simulink model "Marine_LocoMotive_UAV_est_git"  (R2018a)
settings: Solver=ode4  StartTime=0.0  StopTime=40  FixedStep=T  MaxStep=2*T  MinStep=T  RelTol=1e-4
values from neighbouring files (symbols this model uses):
  a_11 = 0.05*m_b    (= 0.625)    [Marine_LocoMotive_UAV_est_git_parameters.m]    (also in Marine_LocoMotive_UAV_medium_est_git_parameters.m = 1.6875; heave_dynamics_chart.m)
  a_33 = m_b    (= 12.5)    [Marine_LocoMotive_UAV_est_git_parameters.m]    (also in Marine_LocoMotive_UAV_medium_est_git_parameters.m = 33.75; heave_dynamics_chart.m)
  A_w = 1*3.3/2    (= 1.65)    [Marine_LocoMotive_UAV_est_git_parameters.m]    (also in Marine_LocoMotive_UAV_medium_est_git_parameters.m = 0.6)
  A_w2 = 1*1.2/2    (= 0.6)    [Marine_LocoMotive_UAV_est_git_parameters.m]    (also in Marine_LocoMotive_UAV_medium_est_git_parameters.m = 0.305)
  Ac = 0.0331    [Marine_LocoMotive_UAV_est_git_parameters.m]    (also in Marine_LocoMotive_UAV_medium_est_git_parameters.m = 0.422)
  alpha_bar = pi/4    (= 0.785398163397)    [Marine_LocoMotive_UAV_est_git_parameters.m]    (also in Marine_LocoMotive_UAV_medium_est_git_parameters.m; heave_dynamics_chart.m = pi/4*sign(V_bar(j)))
  Am = sysd.denominator{1}    [Marine_LocoMotive_UAV_est_git_parameters.m]    (also in Marine_LocoMotive_UAV_medium_est_git_parameters.m)
  Am1_LPF = sysd.denominator{1}    [Marine_LocoMotive_UAV_est_git_parameters.m]    (also in Marine_LocoMotive_UAV_medium_est_git_parameters.m)
  Am2_LPF = sysd.denominator{1}    [Marine_LocoMotive_UAV_est_git_parameters.m]    (also in Marine_LocoMotive_UAV_medium_est_git_parameters.m)
  Am_asw_LPF = sysd.denominator{1}    [Marine_LocoMotive_UAV_est_git_parameters.m]    (also in Marine_LocoMotive_UAV_medium_est_git_parameters.m)
  Am_coup_LPF = sysd.denominator{1}    [Marine_LocoMotive_UAV_est_git_parameters.m]    (also in Marine_LocoMotive_UAV_medium_est_git_parameters.m)
  Am_fast_coup_LPF = sysd.denominator{1}    [Marine_LocoMotive_UAV_est_git_parameters.m]    (also in Marine_LocoMotive_UAV_medium_est_git_parameters.m)
  Am_rdeL_LPF = sysd.denominator{1}    [Marine_LocoMotive_UAV_est_git_parameters.m]    (also in Marine_LocoMotive_UAV_medium_est_git_parameters.m)
  Am_reL_LPF = sysd.denominator{1}    [Marine_LocoMotive_UAV_est_git_parameters.m]    (also in Marine_LocoMotive_UAV_medium_est_git_parameters.m)
  Am_rref20_LPF = sysd.denominator{1}    [Marine_LocoMotive_UAV_est_git_parameters.m]    (also in Marine_LocoMotive_UAV_medium_est_git_parameters.m)
  Am_rref_LPF = sysd.denominator{1}    [Marine_LocoMotive_UAV_est_git_parameters.m]    (also in Marine_LocoMotive_UAV_medium_est_git_parameters.m)
  AmAlpha_LPF = sysd.denominator{1}    [Marine_LocoMotive_UAV_est_git_parameters.m]    (also in Marine_LocoMotive_UAV_medium_est_git_parameters.m)
  Amp_sf = 3    [Marine_LocoMotive_UAV_est_git_parameters.m]    (also in Marine_LocoMotive_UAV_medium_est_git_parameters.m)
  Amp_sf_rp = 0.05*m_u*g    (= 0.8829)    [Marine_LocoMotive_UAV_est_git_parameters.m]    (also in Marine_LocoMotive_UAV_medium_est_git_parameters.m = 9.56475)
  AmV_LPF = sysd.denominator{1}    [Marine_LocoMotive_UAV_est_git_parameters.m]    (also in Marine_LocoMotive_UAV_medium_est_git_parameters.m)
  AmZ_LPF = sysd.denominator{1}    [Marine_LocoMotive_UAV_est_git_parameters.m]    (also in Marine_LocoMotive_UAV_medium_est_git_parameters.m)
  b_11 = 0    [Marine_LocoMotive_UAV_est_git_parameters.m]    (also in Marine_LocoMotive_UAV_medium_est_git_parameters.m; heave_dynamics_chart.m)
  b_33 = 2*m_b*omega_h    (= 19.6349540849)    [Marine_LocoMotive_UAV_est_git_parameters.m]    (also in Marine_LocoMotive_UAV_medium_est_git_parameters.m = 84.8230016469; buoyancy_calc.m = 4.18879020479; heave_dynamics_chart.m = 2*m_b*omega_h)
  Bm = sysd.numerator{1}    [Marine_LocoMotive_UAV_est_git_parameters.m]    (also in Marine_LocoMotive_UAV_medium_est_git_parameters.m)
  Bm1_LPF = sysd.numerator{1}    [Marine_LocoMotive_UAV_est_git_parameters.m]    (also in Marine_LocoMotive_UAV_medium_est_git_parameters.m)
  Bm2_LPF = sysd.numerator{1}    [Marine_LocoMotive_UAV_est_git_parameters.m]    (also in Marine_LocoMotive_UAV_medium_est_git_parameters.m)
  Bm_asw_LPF = sysd.numerator{1}    [Marine_LocoMotive_UAV_est_git_parameters.m]    (also in Marine_LocoMotive_UAV_medium_est_git_parameters.m)
  Bm_coup_LPF = sysd.numerator{1}    [Marine_LocoMotive_UAV_est_git_parameters.m]    (also in Marine_LocoMotive_UAV_medium_est_git_parameters.m)
  Bm_fast_coup_LPF = sysd.numerator{1}    [Marine_LocoMotive_UAV_est_git_parameters.m]    (also in Marine_LocoMotive_UAV_medium_est_git_parameters.m)
  Bm_rdeL_LPF = sysd.numerator{1}    [Marine_LocoMotive_UAV_est_git_parameters.m]    (also in Marine_LocoMotive_UAV_medium_est_git_parameters.m)
  Bm_reL_LPF = sysd.numerator{1}    [Marine_LocoMotive_UAV_est_git_parameters.m]    (also in Marine_LocoMotive_UAV_medium_est_git_parameters.m)
  Bm_rref20_LPF = sysd.numerator{1}    [Marine_LocoMotive_UAV_est_git_parameters.m]    (also in Marine_LocoMotive_UAV_medium_est_git_parameters.m)
  Bm_rref_LPF = sysd.numerator{1}    [Marine_LocoMotive_UAV_est_git_parameters.m]    (also in Marine_LocoMotive_UAV_medium_est_git_parameters.m)
  BmAlpha_LPF = sysd.numerator{1}    [Marine_LocoMotive_UAV_est_git_parameters.m]    (also in Marine_LocoMotive_UAV_medium_est_git_parameters.m)
  BmV_LPF = sysd.numerator{1}    [Marine_LocoMotive_UAV_est_git_parameters.m]    (also in Marine_LocoMotive_UAV_medium_est_git_parameters.m)
  BmZ_LPF = sysd.numerator{1}    [Marine_LocoMotive_UAV_est_git_parameters.m]    (also in Marine_LocoMotive_UAV_medium_est_git_parameters.m)
  C_S = [5;9]*10^-3    [Marine_LocoMotive_UAV_est_git_parameters.m]    (also in Marine_LocoMotive_UAV_medium_est_git_parameters.m; heave_dynamics_chart.m = 0.075/(log10(Re)-2)^2)
  Cd_u = 0.2    [Marine_LocoMotive_UAV_est_git_parameters.m]    (also in Marine_LocoMotive_UAV_medium_est_git_parameters.m)
  D_x = b_11 + D_s(1)    [Marine_LocoMotive_UAV_est_git_parameters.m]    (also in Marine_LocoMotive_UAV_medium_est_git_parameters.m; heave_dynamics_chart.m = b_11 + D_s(i,j))
  D_z = b_33 + D_s(2)    [Marine_LocoMotive_UAV_est_git_parameters.m]    (also in Marine_LocoMotive_UAV_medium_est_git_parameters.m; heave_dynamics_chart.m)
  dc_M_p = 6.7    [Marine_LocoMotive_UAV_est_git_parameters.m]    (also in Marine_LocoMotive_UAV_medium_est_git_parameters.m)
  Delta_h = (A_im/A_b-0.5)*h_b    (= -0.0625)    [Marine_LocoMotive_UAV_est_git_parameters.m]    (also in Marine_LocoMotive_UAV_medium_est_git_parameters.m = -0.075; heave_dynamics_chart.m)
  eps_V = 0.1    [Marine_LocoMotive_UAV_est_git_parameters.m]    (also in Marine_LocoMotive_UAV_medium_est_git_parameters.m)
  epsilon_1 = 5    [Marine_LocoMotive_UAV_est_git_parameters.m]    (also in Marine_LocoMotive_UAV_medium_est_git_parameters.m)
  epsilon_e_u1 = 0.05    [Marine_LocoMotive_UAV_est_git_parameters.m]    (also in Marine_LocoMotive_UAV_medium_est_git_parameters.m)
  epsilon_w = 0    [Marine_LocoMotive_UAV_est_git_parameters.m]    (also in Marine_LocoMotive_UAV_medium_est_git_parameters.m)
  epsilon_w2 = pi    (= 3.14159265359)    [Marine_LocoMotive_UAV_est_git_parameters.m]    (also in Marine_LocoMotive_UAV_medium_est_git_parameters.m)
  g = 9.81    [Marine_LocoMotive_UAV_est_git_parameters.m]    (also in Marine_LocoMotive_UAV_medium_est_git_parameters.m; heave_dynamics_chart.m)
  gamma_d_p = (2*0.3/0.03*2*0.2*12/4)/10    (= 2.4)    [Marine_LocoMotive_UAV_est_git_parameters.m]    (also in Marine_LocoMotive_UAV_medium_est_git_parameters.m)
  H = 10    [Marine_LocoMotive_UAV_est_git_parameters.m]    (also in Marine_LocoMotive_UAV_medium_est_git_parameters.m)
  h_b = 0.25    [Marine_LocoMotive_UAV_est_git_parameters.m]    (also in Marine_LocoMotive_UAV_medium_est_git_parameters.m = 0.3; buoyancy_calc.m = 0.15; heave_dynamics_chart.m)
  J_b = m_b*h_b*l_b/12    (= 0.208333333333)    [Marine_LocoMotive_UAV_est_git_parameters.m]    (also in Marine_LocoMotive_UAV_medium_est_git_parameters.m = 1.265625; heave_dynamics_chart.m)
  J_u = 0.03    [Marine_LocoMotive_UAV_est_git_parameters.m]    (also in Marine_LocoMotive_UAV_medium_est_git_parameters.m = 1.51708333333)
  K = 40    [Marine_LocoMotive_UAV_est_git_parameters.m]    (also in Marine_LocoMotive_UAV_medium_est_git_parameters.m = 83.3333333333)
  k3 = 24    [Marine_LocoMotive_UAV_est_git_parameters.m]    (also in Marine_LocoMotive_UAV_medium_est_git_parameters.m)
  k4 = 0.8    [Marine_LocoMotive_UAV_est_git_parameters.m]    (also in Marine_LocoMotive_UAV_medium_est_git_parameters.m)
  k_w = omega_w^2/g    (= 0.0628797426165)    [Marine_LocoMotive_UAV_est_git_parameters.m]    (also in Marine_LocoMotive_UAV_medium_est_git_parameters.m = 0.160972141098; heave_dynamics_chart.m = omega_w^2/g)
  k_w2 = omega_w2^2/g    (= 0.160972141098)    [Marine_LocoMotive_UAV_est_git_parameters.m]    (also in Marine_LocoMotive_UAV_medium_est_git_parameters.m = 0.251518970466)
  kd_a = 5.6    [Marine_LocoMotive_UAV_est_git_parameters.m]    (also in Marine_LocoMotive_UAV_medium_est_git_parameters.m)
  kd_r = 19.5    [Marine_LocoMotive_UAV_est_git_parameters.m]    (also in Marine_LocoMotive_UAV_medium_est_git_parameters.m)
  kd_t = 10    [Marine_LocoMotive_UAV_est_git_parameters.m]    (also in Marine_LocoMotive_UAV_medium_est_git_parameters.m = 25)
  kd_x = 5    [Marine_LocoMotive_UAV_est_git_parameters.m]    (also in Marine_LocoMotive_UAV_medium_est_git_parameters.m)
  kd_z = 2    [Marine_LocoMotive_UAV_est_git_parameters.m]    (also in Marine_LocoMotive_UAV_medium_est_git_parameters.m)
  ki_a = 1.6    [Marine_LocoMotive_UAV_est_git_parameters.m]    (also in Marine_LocoMotive_UAV_medium_est_git_parameters.m)
  ki_r = 9    [Marine_LocoMotive_UAV_est_git_parameters.m]    (also in Marine_LocoMotive_UAV_medium_est_git_parameters.m)
  ki_T = 12    [Marine_LocoMotive_UAV_est_git_parameters.m]    (also in Marine_LocoMotive_UAV_medium_est_git_parameters.m)
  ki_x = 1.2    [Marine_LocoMotive_UAV_est_git_parameters.m]    (also in Marine_LocoMotive_UAV_medium_est_git_parameters.m)
  ki_z = 1    [Marine_LocoMotive_UAV_est_git_parameters.m]    (also in Marine_LocoMotive_UAV_medium_est_git_parameters.m)
  kp_a = 9.6    [Marine_LocoMotive_UAV_est_git_parameters.m]    (also in Marine_LocoMotive_UAV_medium_est_git_parameters.m)
  kp_r = 45    [Marine_LocoMotive_UAV_est_git_parameters.m]    (also in Marine_LocoMotive_UAV_medium_est_git_parameters.m)
  kp_t = 20    [Marine_LocoMotive_UAV_est_git_parameters.m]    (also in Marine_LocoMotive_UAV_medium_est_git_parameters.m = 50)
  kp_T = 25    [Marine_LocoMotive_UAV_est_git_parameters.m]    (also in Marine_LocoMotive_UAV_medium_est_git_parameters.m)
  kp_x = 7    [Marine_LocoMotive_UAV_est_git_parameters.m]    (also in Marine_LocoMotive_UAV_medium_est_git_parameters.m)
  kp_z = 3    [Marine_LocoMotive_UAV_est_git_parameters.m]    (also in Marine_LocoMotive_UAV_medium_est_git_parameters.m)
  L = 0.2    [Marine_LocoMotive_UAV_est_git_parameters.m]    (also in Marine_LocoMotive_UAV_medium_est_git_parameters.m = 0.8)
  l_b = 0.8    [Marine_LocoMotive_UAV_est_git_parameters.m]    (also in Marine_LocoMotive_UAV_medium_est_git_parameters.m = 1.5; buoyancy_calc.m = 0.5; heave_dynamics_chart.m)
  Lc_0 = 7    [Marine_LocoMotive_UAV_est_git_parameters.m]    (also in Marine_LocoMotive_UAV_medium_est_git_parameters.m = 20)
  LIMIT_CMD_PITCH = 45*pi/180    (= 0.785398163397)    [Marine_LocoMotive_UAV_est_git_parameters.m]    (also in Marine_LocoMotive_UAV_medium_est_git_parameters.m)
  LIMIT_uCMD_HEIGHT = 0.9*n_motors*K    (= 144)    [Marine_LocoMotive_UAV_est_git_parameters.m]    (also in Marine_LocoMotive_UAV_medium_est_git_parameters.m = 450)
  m_b = rho_w*Vol_b/4    (= 12.5)    [Marine_LocoMotive_UAV_est_git_parameters.m]    (also in Marine_LocoMotive_UAV_medium_est_git_parameters.m = 33.75; buoyancy_calc.m = 5; heave_dynamics_chart.m)
  m_u = 1.8    [Marine_LocoMotive_UAV_est_git_parameters.m]    (also in Marine_LocoMotive_UAV_medium_est_git_parameters.m = 19.5)
  min_sf = 5    [Marine_LocoMotive_UAV_est_git_parameters.m]    (also in Marine_LocoMotive_UAV_medium_est_git_parameters.m)
  min_sf_rp = 0.35*m_u*g    (= 6.1803)    [Marine_LocoMotive_UAV_est_git_parameters.m]    (also in Marine_LocoMotive_UAV_medium_est_git_parameters.m = 66.95325)
  n_motors = 4    [Marine_LocoMotive_UAV_est_git_parameters.m]    (also in Marine_LocoMotive_UAV_medium_est_git_parameters.m = 6)
  nu_w = 1.787*10^-6    (= 1.787e-06)    [Marine_LocoMotive_UAV_est_git_parameters.m]    (also in Marine_LocoMotive_UAV_medium_est_git_parameters.m; buoyancy_calc.m; heave_dynamics_chart.m)
  omega_w = 2*pi/T_w    (= 0.785398163397)    [Marine_LocoMotive_UAV_est_git_parameters.m]    (also in Marine_LocoMotive_UAV_medium_est_git_parameters.m = 1.25663706144; heave_dynamics_chart.m = 2*pi/T_i)
  omega_w2 = 2*pi/T_w2    (= 1.25663706144)    [Marine_LocoMotive_UAV_est_git_parameters.m]    (also in Marine_LocoMotive_UAV_medium_est_git_parameters.m = 1.57079632679)
  r_0 = sqrt( (X0_b(1) - X0_u(1))^2 +(X0_b(2) - X0_u(2))^2 )    [Marine_LocoMotive_UAV_est_git_parameters.m]    (also in Marine_LocoMotive_UAV_medium_est_git_parameters.m)
  R_b = 0.1    [buoyancy_calc.m]
  r_bar = Lc_0-0.3    (= 6.7)    [Marine_LocoMotive_UAV_est_git_parameters.m]    (also in Marine_LocoMotive_UAV_medium_est_git_parameters.m = 19.7)
  r_min = (zu_bar-H)-0.2    [Marine_LocoMotive_UAV_est_git_parameters.m]    (also in Marine_LocoMotive_UAV_medium_est_git_parameters.m)
  rho_a = 1.225    [Marine_LocoMotive_UAV_est_git_parameters.m]    (also in Marine_LocoMotive_UAV_medium_est_git_parameters.m)
  rho_w = 1000    [Marine_LocoMotive_UAV_est_git_parameters.m]    (also in Marine_LocoMotive_UAV_medium_est_git_parameters.m; buoyancy_calc.m; heave_dynamics_chart.m)
  T = 1/500    (= 0.002)    [Marine_LocoMotive_UAV_est_git_parameters.m]    (also in Marine_LocoMotive_UAV_medium_est_git_parameters.m)
  T_init = 10    [Marine_LocoMotive_UAV_est_git_parameters.m]    (also in Marine_LocoMotive_UAV_medium_est_git_parameters.m)
  Theta0 = 0    [Marine_LocoMotive_UAV_est_git_parameters.m]    (also in Marine_LocoMotive_UAV_medium_est_git_parameters.m)
  torque_corr = 2*cosd(60)+1    [Marine_LocoMotive_UAV_est_git_parameters.m]    (also in Marine_LocoMotive_UAV_medium_est_git_parameters.m)
  u_s = w_dir*A_w^2*omega_w*k_w*exp(2*k_w*(-Delta_h/2))    [Marine_LocoMotive_UAV_est_git_parameters.m]    (also in Marine_LocoMotive_UAV_medium_est_git_parameters.m)
  u_s2 = w_dir2*A_w2^2*omega_w2*k_w2*exp(2*k_w2*(-Delta_h/2))    [Marine_LocoMotive_UAV_est_git_parameters.m]    (also in Marine_LocoMotive_UAV_medium_est_git_parameters.m)
  u_t = -1*0.5*1    (= -0.5)    [Marine_LocoMotive_UAV_est_git_parameters.m]    (also in Marine_LocoMotive_UAV_medium_est_git_parameters.m)
  u_w = 0*0.2    (= 0)    [Marine_LocoMotive_UAV_est_git_parameters.m]    (also in Marine_LocoMotive_UAV_medium_est_git_parameters.m)
  V0_b = [u_t+u_w+u_s+v_x_w, v_z_w].*[1 1]    [Marine_LocoMotive_UAV_est_git_parameters.m]    (also in Marine_LocoMotive_UAV_medium_est_git_parameters.m = [u_t+u_w+u_s+v_x_w, v_z_w])
  V0_u = V0_b    [Marine_LocoMotive_UAV_est_git_parameters.m]    (also in Marine_LocoMotive_UAV_medium_est_git_parameters.m = [0 0])
  V_bar = 4    [Marine_LocoMotive_UAV_est_git_parameters.m]    (also in Marine_LocoMotive_UAV_medium_est_git_parameters.m; heave_dynamics_chart.m = [-20:0.1:20]')
  Vol_b = A_b*l_b    (= 0.05)    [Marine_LocoMotive_UAV_est_git_parameters.m]    (also in Marine_LocoMotive_UAV_medium_est_git_parameters.m = 0.135; heave_dynamics_chart.m)
  w_dir = 1    [Marine_LocoMotive_UAV_est_git_parameters.m]    (also in Marine_LocoMotive_UAV_medium_est_git_parameters.m; heave_dynamics_chart.m)
  w_dir2 = 1    [Marine_LocoMotive_UAV_est_git_parameters.m]    (also in Marine_LocoMotive_UAV_medium_est_git_parameters.m)
  X0_b = [0,H-Delta_h]    [Marine_LocoMotive_UAV_est_git_parameters.m]    (also in Marine_LocoMotive_UAV_medium_est_git_parameters.m)
  X0_u = X0_b + [3/7 3/7]*Lc_0    [Marine_LocoMotive_UAV_est_git_parameters.m]    (also in Marine_LocoMotive_UAV_medium_est_git_parameters.m)
  zu_bar = X0_b(2) + Lc_0*sin(alpha_bar_0)    [Marine_LocoMotive_UAV_est_git_parameters.m]    (also in Marine_LocoMotive_UAV_medium_est_git_parameters.m)
undefined symbols (not defined in the file or in its folder): Am_HPF, Am_LPF, Am_LPF2, an1, an1_v, an2, an3, Bm_HPF, Bm_LPF, Bm_LPF2, bn1, bn1_v, bn2, bn3, DiscIntNeverNeededParam, F, Light, magnitude, MIL, OMEGA_FILTER_OUTER, Tc, Tg, Tn, Ts, Tsc, Tz, X_GPS_offset
libraries: simulink x55, simulink_extras x9, aerolibwind2 x2
(part 1 of 9)
settings Model: Creator=Ahmad  LastModifiedBy=Ahmad
settings SolverCC: InitialStep=T  AlgebraicLoopSolver=LineSearch

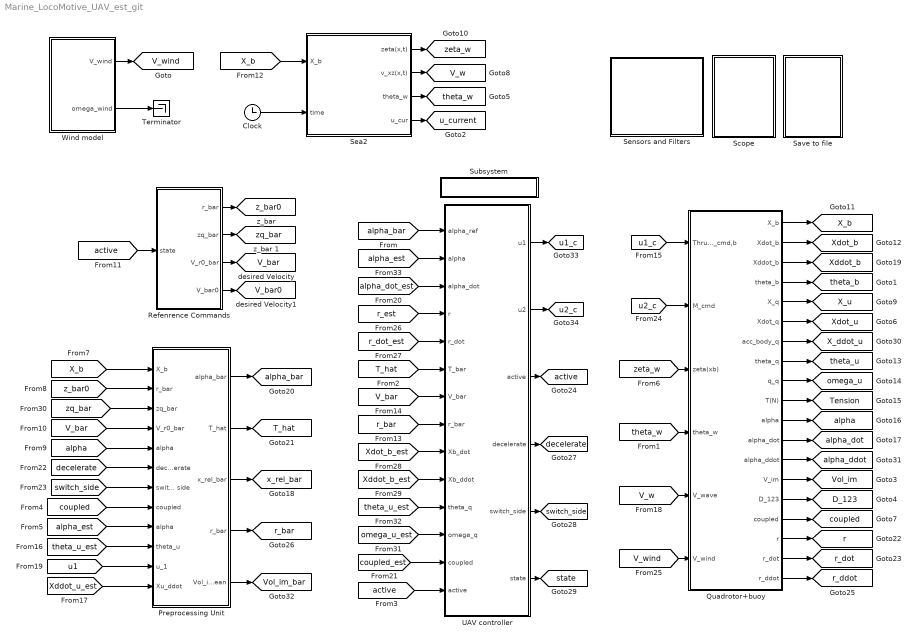
== system Marine_LocoMotive_UAV_est_git ==
  Clock : Clock
  Preprocessing Unit : Subsystem
  Quadrotor+buoy : Subsystem
  Refenrence Commands : Subsystem
  Save to file : Subsystem
  Scope : Subsystem
  Sea2 : Subsystem
  Sensors and Filters : Subsystem
  Subsystem : Subsystem
      settings: OpenFcn=Marine_LocoMotive_UAV_est_parameters
      mask Display:
      | text(.5,.5,'load parameters',...
      | 	'horizontalalignment','center');
  Terminator : Terminator
  UAV controller : Subsystem
  Wind model : Subsystem
  tag scope: D_123=global, T_hat=global, Tension=global, V_bar0=global, V_bar=global, V_w=global, V_wind=global, Vol_im=global, Vol_im_bar=global, X_b=global, X_ddot_u=global, X_u=global, Xddot_b=global, Xdot_b=global, Xdot_u=global, active=global, alpha=global, alpha_bar=global, alpha_ddot=global, alpha_dot=global, coupled=global, decelerate=global, omega_u=global, r=global, r_bar=global, r_ddot=global, r_dot=global, state=global, switch_side=global, theta_b=global, theta_u=global, theta_w=global, u1_c=global, u2_c=global, u_current=global, x_rel_bar=global, z_bar0=global, zeta_w=global, zq_bar=global
  wires:
  Clock/1 -> Sea2/2(time)
  [X_b] -> Sea2/1(X_b)
  Sea2/1(zeta(x,t)) -> [zeta_w]
  Sea2/2(v_xz(x,t)) -> [V_w]
  Sea2/3(theta_w) -> [theta_w]
  [theta_w] -> Quadrotor+buoy/4(theta_w)
  [V_w] -> Quadrotor+buoy/5(V_wave)
  [zeta_w] -> Quadrotor+buoy/3(zeta(xb))
  Quadrotor+buoy/5(X_q) -> [X_u]
  Quadrotor+buoy/1(X_b) -> [X_b]
  Quadrotor+buoy/2(Xdot_b) -> [Xdot_b]
  Quadrotor+buoy/8(theta_q) -> [theta_u]
  Quadrotor+buoy/9(q_q) -> [omega_u]
  Quadrotor+buoy/10(T(N)) -> [Tension]
  Quadrotor+buoy/11(alpha) -> [alpha]
  Quadrotor+buoy/12(alpha_dot) -> [alpha_dot]
  [X_b] -> Preprocessing Unit/1(X_b)
  Preprocessing Unit/1(alpha_bar) -> [alpha_bar]
  Preprocessing Unit/2(T_hat) -> [T_hat]
  Quadrotor+buoy/3(Xddot_b) -> [Xddot_b]
  Quadrotor+buoy/4(theta_b) -> [theta_b]
  Quadrotor+buoy/6(Xdot_q) -> [Xdot_u]
  Sea2/4(u_cur) -> [u_current]
  Quadrotor+buoy/14(V_im) -> [Vol_im]
  Quadrotor+buoy/15(D_123) -> [D_123]
  [alpha_bar] -> UAV controller/1(alpha_ref)
  [alpha_est] -> UAV controller/2(alpha)
  [alpha_dot_est] -> UAV controller/3(alpha_dot)
  [T_hat] -> UAV controller/6(T_bar)
  [V_bar] -> UAV controller/7(V_bar)
  [Xdot_b_est] -> UAV controller/9(Xb_dot)
  [Xddot_b_est] -> UAV controller/10(Xb_ddot)
  [theta_u_est] -> UAV controller/11(theta_q)
  [omega_u_est] -> UAV controller/12(omega_q)
  Quadrotor+buoy/16(coupled) -> [coupled]
  [active] -> Refenrence Commands/1(state)
  Preprocessing Unit/3(x_rel_bar) -> [x_rel_bar]
  [r_bar] -> UAV controller/8(r_bar)
  Quadrotor+buoy/17(r) -> [r]
  Quadrotor+buoy/18(r_dot) -> [r_dot]
  [r_est] -> UAV controller/4(r)
  UAV controller/3(" active") -> [active]
  [active] -> UAV controller/14(active)
  [coupled_est] -> UAV controller/13(coupled)
  Quadrotor+buoy/19(r_ddot) -> [r_ddot]
  [r_dot_est] -> UAV controller/5(r_dot)
  Preprocessing Unit/4(" r_bar") -> [r_bar]
  UAV controller/4(" decelerate") -> [decelerate]
  [decelerate] -> Preprocessing Unit/6(decelerate)
  UAV controller/5(" switch_side") -> [switch_side]
  UAV controller/6(state) -> [state]
  [switch_side] -> Preprocessing Unit/7(switch side)
  [alpha] -> Preprocessing Unit/5(alpha)
  [coupled] -> Preprocessing Unit/8(coupled)
  Quadrotor+buoy/7(acc_body_q) -> [X_ddot_u]
  Quadrotor+buoy/13(alpha_ddot) -> [alpha_ddot]
  [u1] -> Preprocessing Unit/11("u_1 ")
  [alpha_est] -> Preprocessing Unit/9("alpha ")
  [theta_u_est] -> Preprocessing Unit/10("theta_u ")
  [Xddot_u_est] -> Preprocessing Unit/12(Xu_ddot)
  Preprocessing Unit/5(Vol_im_mean) -> [Vol_im_bar]
  Wind model/1(V_wind) -> [V_wind]
  Wind model/2(omega_wind) -> Terminator/1
  [V_wind] -> Quadrotor+buoy/6(V_wind)
  Refenrence Commands/1(r_bar) -> [z_bar0]
  [z_bar0] -> Preprocessing Unit/2(r_bar)
  Refenrence Commands/4(V_bar0) -> [V_bar0]
  Refenrence Commands/3(V_r0_bar) -> [V_bar]
  [V_bar] -> Preprocessing Unit/4(V_r0_bar)
  UAV controller/1(u1) -> [u1_c]
  UAV controller/2(u2) -> [u2_c]
  [u1_c] -> Quadrotor+buoy/1(Thrust_cmd,b)
  [u2_c] -> Quadrotor+buoy/2(M_cmd)
  Refenrence Commands/2(zq_bar) -> [zq_bar]
  [zq_bar] -> Preprocessing Unit/3(zq_bar)

== system Marine_LocoMotive_UAV_est_git/Preprocessing Unit ==
  X_b : Inport
  r_bar : Inport  Port=2
  zq_bar : Inport  Port=3
  V_r0_bar : Inport  Port=4
  alpha : Inport  Port=5
  decelerate : Inport  Port=6
  switch side : Inport  Port=7
  coupled : Inport  Port=8
  "alpha " : Inport  Port=9
  "theta_u " : Inport  Port=10
  "u_1 " : Inport  Port=11
  Xu_ddot : Inport  Port=12
  Alpha_bar : Subsystem
  Buoy immersed volume estimation : Subsystem
  Discrete Transfer Fcn1 : DiscreteTransferFcn  Numerator=BmZ_LPF  Denominator=AmZ_LPF  InitialStates=[1 1]*(1-sum(AmZ_LPF))/(sum(BmZ_LPF))*X0_b(2)
  Mux : Mux  Inputs=3
  Sum : Sum  Inputs=|+-
  "T_bar " : Subsystem
  Terminator : Terminator
  "Theta_bar " : Subsystem
  V_r0_bar1 : InportShadow  Port=4
  buoy elvation : Scope
  r_bar1 : InportShadow  Port=2
  switch side1 : InportShadow  Port=7
  z_b : Selector  InputPortWidth=2  IndexOptions=Index vector (dialog)  Indices=2  OutputSizes=1
  alpha_bar : Outport
  T_hat : Outport  Port=2
  x_rel_bar : Outport  Port=3
  " r_bar" : Outport  Port=4
  Vol_im_mean : Outport  Port=5
  tag scope: T_bar=global, T_est=global, theta_bar=global, z_bar=global
  wires:
  X_b/1 -> z_b/1
  "Theta_bar "/1(theta_bar) -> "T_bar "/2(theta_bar), [theta_bar]
  V_r0_bar/1 -> "Theta_bar "/2(V_r0_bar)
  zq_bar/1 -> Alpha_bar/3(zq_bar)
  Mux/1 -> buoy elvation/1
  Sum/1 -> Mux/3
  z_b/1 -> Discrete Transfer Fcn1/1, Mux/1, Sum/1
  Discrete Transfer Fcn1/1 -> Mux/2, Sum/2, Alpha_bar/1(zb)  "better"
  [D11_bar] -> "Theta_bar "/3(D11_bar)
  Alpha_bar/1(alpha_bar) -> alpha_bar/1, "T_bar "/1("alpha_bar "), "Theta_bar "/1("alpha_bar ")
  "T_bar "/1(T_hat) -> T_hat/1
  "T_bar "/2(T_bar) -> [T_bar]
  r_bar/1 -> Alpha_bar/2(r_bar)
  Alpha_bar/2(x_rel_bar) -> x_rel_bar/1
  alpha/1 -> Alpha_bar/4(alpha)
  decelerate/1 -> Alpha_bar/5(decelerate)
  switch side/1 -> Alpha_bar/6(switch side)
  coupled/1 -> "T_bar "/4(coupled)
  switch side1/1 -> "Theta_bar "/4(switch side1)
  "theta_u "/1 -> "T_bar "/6(theta_u)
  "u_1 "/1 -> "T_bar "/7(u1)
  Xu_ddot/1 -> "T_bar "/8(Xu_ddot)
  "alpha "/1 -> "T_bar "/5(alpha)
  "T_bar "/3(T_est) -> [T_est]
  Alpha_bar/3(z_bar) -> [z_bar]
  Buoy immersed volume estimation/2(Vol_im_mean) -> Vol_im_mean/1
  V_r0_bar1/1 -> "T_bar "/3(V_r0_bar)
  r_bar1/1 -> " r_bar"/1
  Buoy immersed volume estimation/1(Vol_im_expected) -> Terminator/1
  "T_bar "/4(D_11_bar) -> [D11_bar]

== system Marine_LocoMotive_UAV_est_git/Quadrotor+buoy ==
  Thrust_cmd,b : Inport
  M_cmd : Inport  Port=2
  zeta(xb) : Inport  Port=3
  theta_w : Inport  Port=4
  V_wave : Inport  Port=5
  V_wind : Inport  Port=6
  3-DOF equations of motion Earth frame : Subsystem  mask(3DOF EoM, earth frame){pos_b_ini=X0_b, pos_u_ini=X0_u, theta_b_ini=0, alpha_0=alpha_bar, v_b_ini=V0_b, v_u_ini=V0_u, theta_q_ini=Theta0, q_b_ini=0, m_u=m_u, J_u=J_u, m_b=m_b, J_b=J_b, a_ii=[a_11 a_33], b_ii=[D_x,D_z], L=Lc_0, g=g, coupled_ini=off}
      mask prompts: pos_b_ini "Buoy initial position (x z):"; pos_u_ini "UAV initial position (x z):"; theta_b_ini "Buoy initial body attitude (quadrotor):"; alpha_0 "Cable initial angle:"; v_b_ini "Buoy initial velocity (x z):"; v_u_ini "UAV initial velocity (x z):"; theta_q_ini "Quadrotor initial body attitude (quadrotor):"; q_b_ini "Quadrotor initial body rotation rate:"; m_u "Quadrotor mass:"; J_u "Quadrotor moment of Inertia:"; m_b "Buoy mass:"; J_b "Buoy moment of Inertia:"; a_ii "Added mass (1x3):"; b_ii "Buoy damping coefficients (1x2):"; L "Cable length:"; g "gravity:"; coupled_ini "Initial coupling state (checked for coupled)"
      mask Display:
      | port_label('input',1,'u_1 (N)','texmode','on');
      | port_label('input',2,'u_2 (N.m)','texmode','on');
      | port_label('input',3,'\zeta (m)','texmode','on');
      | port_label('input',4,'\theta_w (rad)','texmode','on');
      | port_label('input',5,'V_{wave} (m/s)','texmode','on');
      | port_label('input',6,'V_{wind} (m/s)','texmode','on');
      | 
      | port_label('output',1,'X_b (m)','texmode','on');
      | port_label('output',2,'X_{b,dot} (m/s)','texmode','on');
      | port_label('output',3,'X_{b,ddot} (m/s)','texmode','on');
      | port_label('output',4,'\theta_b(rad)','texmode','on');
      | port_label('output',5,'X_q (m)','texmode','on');
      | port_label('output',6,'X_{q,dot} (m/s)','texmode','on');
      | port_label('output',7,'X_{q,ddot} (m/s^2)','texmode','on');
      | port_label('output',8,'\theta_q(rad)','texmode','on');
      | port_label('output',9,'\omega_q (rad/s)','texmode','on');
      | port_label('output',10,'\alpha (rad)','texmode','on');
      | port_label('output',11,'\alpha_{dot} (rad/s)','texmode','on');
      | port_label('output',12,'\alpha_{ddot} (rad/s)','texmode','on');
      | port_label('output',13,'r (m)','texmode','on');
      | port_label('output',14,'r_{dot} (m/s)','texmode','on');
      | port_label('output',15,'r_{ddot} (m/s)','texmode','on');
      | port_label('output',16,'T (N)','texmode','on');
      | port_label('output',17,'V_{im} (m^3)','texmode','on');
      | port_label('output',18,'D_{123}','texmode','on');
      | port_label('output',19,'coupled','texmode','on');
  Gain : Gain
  Gain1 : Gain
  Mux : Mux  Inputs=2
  Mux1 : Mux  Inputs=2
  Saturation - Limit Height Controller1 : Saturate  UpperLimit=K*L*torque_corr  LowerLimit=-K*L*torque_corr
  Saturation - Limit Height Controller3 : Saturate  UpperLimit=n_motors*K  LowerLimit=0
  Torque : Scope
  "Xb " : Scope
  "Xq " : Scope
  motor dynamics (thrust) : DiscreteTransferFcn  Numerator=Bm  Denominator=Am  InitialStates=-Am(2)/Bm(2)*m_u*g/cos(Theta0)
  motor dynamics (torque) : DiscreteTransferFcn  Numerator=Bm  Denominator=Am
  thrust : Scope
  X_b : Outport
  Xdot_b : Outport  Port=2
  Xddot_b : Outport  Port=3
  theta_b : Outport  Port=4
  X_q : Outport  Port=5
  Xdot_q : Outport  Port=6
  acc_body_q : Outport  Port=7
  theta_q : Outport  Port=8
  q_q : Outport  Port=9
  T(N) : Outport  Port=10
  alpha : Outport  Port=11
  alpha_dot : Outport  Port=12
  alpha_ddot : Outport  Port=13
  V_im : Outport  Port=14
  D_123 : Outport  Port=15
  coupled : Outport  Port=16
  r : Outport  Port=17
  r_dot : Outport  Port=18
  r_ddot : Outport  Port=19
  tag scope: u1=global, u2=global
  wires:
  Saturation - Limit Height Controller3/1 -> Gain/1, Mux/2
  motor dynamics (torque)/1 -> Saturation - Limit Height Controller1/1
  M_cmd/1 -> Mux1/1, motor dynamics (torque)/1
  Thrust_cmd,b/1 -> Mux/1, motor dynamics (thrust)/1
  Saturation - Limit Height Controller1/1 -> Mux1/2, Gain1/1
  zeta(xb)/1 -> 3-DOF equations of motion Earth frame/3(zeta)
  theta_w/1 -> 3-DOF equations of motion Earth frame/4(theta_w)
  V_wave/1 -> 3-DOF equations of motion Earth frame/5(V_w)
  3-DOF equations of motion Earth frame/5(Xu) -> "Xq "/1, X_q/1  "X_q"
  3-DOF equations of motion Earth frame/1(Xb) -> "Xb "/1, X_b/1  "X_b"
  3-DOF equations of motion Earth frame/2(Xb_dot) -> Xdot_b/1  "Xdot_b"
  3-DOF equations of motion Earth frame/6(Xu_dot) -> Xdot_q/1  "V_q"
  3-DOF equations of motion Earth frame/4(Attitude_buoy) -> theta_b/1  "theta_b"
  3-DOF equations of motion Earth frame/8(Attitude_quadrotor) -> theta_q/1  "theta_q"
  3-DOF equations of motion Earth frame/9(q_quadrotor) -> q_q/1  "omega_q"
  3-DOF equations of motion Earth frame/3(Xb_ddot) -> Xddot_b/1
  motor dynamics (thrust)/1 -> Saturation - Limit Height Controller3/1
  3-DOF equations of motion Earth frame/11(alpha_dot) -> alpha_dot/1  "alpha_dot"
  3-DOF equations of motion Earth frame/16(Cable Tension) -> T(N)/1  "tension"
  3-DOF equations of motion Earth frame/10(alpha) -> alpha/1  "alpha"
  Mux/1 -> thrust/1
  Mux1/1 -> Torque/1
  3-DOF equations of motion Earth frame/17(V_im) -> V_im/1
  Gain/1 -> 3-DOF equations of motion Earth frame/1(u1), [u1]
  Gain1/1 -> [u2], 3-DOF equations of motion Earth frame/2(u2)
  3-DOF equations of motion Earth frame/18("D_123 ") -> D_123/1
  3-DOF equations of motion Earth frame/19(coupled) -> coupled/1
  3-DOF equations of motion Earth frame/13("  r") -> r/1
  3-DOF equations of motion Earth frame/14("  rdot") -> r_dot/1
  3-DOF equations of motion Earth frame/15("  rddot") -> r_ddot/1
  3-DOF equations of motion Earth frame/7(Xu_ddot) -> acc_body_q/1
  3-DOF equations of motion Earth frame/12(alpha_ddot) -> alpha_ddot/1
  V_wind/1 -> 3-DOF equations of motion Earth frame/6(V_wind)

== system Marine_LocoMotive_UAV_est_git/Refenrence Commands ==
  note: Smooth reference signals
  note: Initialization phase, reference r and zu
  note: Saturation protection
  note: V_r0_bar is the velocity of the buoy relative
      | to the water current (wave velocity is not included)
  note: Refecence velocity
  state : Inport
  "  Vbar  " : Scope
  "  c" : Scope
  Bias : Bias  Bias=H+h_b/2
  Bias1 : Bias  Bias=-H-h_b/2
  Constant : Constant  Value=H
  Discrete Transfer Fcn (with initial outputs)1 : simulink_extras/Additional Discrete/Discrete Transfer Fcn (with initial outputs)  N=Bm_rref_LPF  D=Am_rref_LPF  U0=0  Y0=r_0  TS=-1
      settings: SourceProductName=Simulink  SourceProductBaseCode=SL
  Discrete Transfer Fcn (with initial outputs)3 : simulink_extras/Additional Discrete/Discrete Transfer Fcn (with initial outputs)  N=BmV_LPF  D=AmV_LPF  U0=0  Y0=0  TS=-1
      settings: SourceProductName=Simulink  SourceProductBaseCode=SL
  Discrete Transfer Fcn (with initial outputs)4 : simulink_extras/Additional Discrete/Discrete Transfer Fcn (with initial outputs)  N=Bm_rref20_LPF  D=Am_rref20_LPF  U0=0  Y0=r_0  TS=-1
      settings: SourceProductName=Simulink  SourceProductBaseCode=SL
  From File : FromFile  Commented=on  FileName=Export\with waves\SVC\V_bar.mat  SampleTime=0
  From File1 : FromFile  Commented=on  FileName=Export\no waves\SVC\V_bar.mat  SampleTime=0
  From File2 : FromFile  FileName=Export\Monte Carlo\CM_21\SVCS\V_bar.mat  SampleTime=0
  Gain : Gain  Gain=0
  Manual Switch1 : ManualSwitch  CurrentSetting=0
  Manual Switch2 : ManualSwitch  Commented=on
  Manual Switch3 : ManualSwitch
  Manual Switch4 : ManualSwitch
  Mux3 : Mux  Inputs=3
  "Rate Limiter for fly over test " : RateLimiter  RisingSlewLimit=2.5/10  FallingSlewLimit=-2.5/10  SampleTimeMode=inherited
  Saturation Dynamic : simulink/Discontinuities/Saturation Dynamic  OutMin=[]  OutMax=[]  OutDataTypeStr=Inherit: Same as second input  OutDataType=fixdt(1, 16)  OutScaling=2^-10  DoSatur=off
  Saturation Dynamic1 : simulink/Discontinuities/Saturation Dynamic  OutMin=[]  OutMax=[]  OutDataTypeStr=Inherit: Same as second input  OutDataType=fixdt(1, 16)  OutScaling=2^-10  DoSatur=off
  Selector1 : Selector  InputPortWidth=2  IndexOptions=Index vector (dialog)  Indices=1  OutputSizes=1
  Step : Step  Time=T_init  After=V_bar+1  SampleTime=0
  Step1 : Step  Time=T_init+25  After=V_bar+1  SampleTime=0
  Step3 : Step  Time=T_init+25+20  After=V_bar  SampleTime=0
  Step5 : Step  Commented=on  Time=T_init+20  After=-20  SampleTime=0
  Step6 : Step  Time=T_init  After=20  SampleTime=0
  Sum : Sum  Inputs=+--
  Sum2 : Sum  Inputs=|++
  Switch{,1..2,4} (4 alike) : Switch  Criteria=u2 > Threshold
  cable length : Constant  Value=Lc_0
  initialize : Step  SampleTime=0
  initialize r_bar : Step  Time=20  SampleTime=0
  minimum velocity error : Constant
  r error threshold [m] : Constant  Value=0.05
  r_bar_0 : Constant  Value=r_0
  "r_ref " : Constant  Value=r_bar
  r_ref for the coupled case (pulling) : Constant  Value=Lc_0
  setpoint velocity controller : MATLAB Function  TreatAsAtomicUnit=on
  smooth z_bar : simulink_extras/Additional Discrete/Discrete Transfer Fcn (with initial outputs)  N=Bm_rref_LPF  D=Am_rref_LPF  U0=X0_u(2)-0.015  Y0=X0_u(2)-0.015  TS=-1
      settings: SourceProductName=Simulink  SourceProductBaseCode=SL
  z_ref : Constant  Value=zu_bar
  zu_bar_0 : Constant  Value=X0_u(2)-0.015
  r_bar : Outport
  zq_bar : Outport  Port=2
  V_r0_bar : Outport  Port=3
  V_bar0 : Outport  Port=4
  wires:
  Step/1 -> Sum/1
  Step1/1 -> Sum/2
  Manual Switch3/1 -> Mux3/3, setpoint velocity controller/5(V0_bar), V_bar0/1
  r_ref for the coupled case (pulling)/1 -> Switch/1, Saturation Dynamic1/1
  Switch1/1 -> Switch/3  "r_ref when not 'pulling'"
  state/1 -> Switch/2
  Saturation Dynamic/1 -> zq_bar/1, Bias1/1
  Constant/1 -> Saturation Dynamic/3
  Bias/1 -> Saturation Dynamic/1
  Saturation Dynamic1/1 -> r_bar/1
  Bias1/1 -> Saturation Dynamic1/3
  smooth z_bar/1 -> Saturation Dynamic/2
  Switch4/1 -> Bias/1, Saturation Dynamic1/2  "r_bar"
  r_bar_0/1 -> Switch1/3
  "r_ref "/1 -> Switch1/1
  zu_bar_0/1 -> Switch2/3
  initialize/1 -> Switch1/2, Switch2/2
  z_ref/1 -> Switch2/1
  Switch2/1 -> smooth z_bar/1
  Switch/1 -> Discrete Transfer Fcn (with initial outputs)1/1, Discrete Transfer Fcn (with initial outputs)4/1
  Step3/1 -> Sum/3
  minimum velocity error/1 -> setpoint velocity controller/1(eps)
  [r_est] -> setpoint velocity controller/2(r)
  r error threshold [m]/1 -> setpoint velocity controller/3(er_thr)
  cable length/1 -> setpoint velocity controller/4(Lc0)
  Selector1/1 -> setpoint velocity controller/6(V)
  [Xdot_b_est] -> Selector1/1
  setpoint velocity controller/2(c) -> "  c"/1
  Discrete Transfer Fcn (with initial outputs)3/1 -> Manual Switch1/2, Mux3/1
  Mux3/1 -> "  Vbar  "/1
  initialize r_bar/1 -> Switch4/2
  Discrete Transfer Fcn (with initial outputs)4/1 -> Switch4/1
  Discrete Transfer Fcn (with initial outputs)1/1 -> Switch4/3
  Manual Switch1/1 -> V_r0_bar/1
  From File/1 -> Manual Switch2/2
  From File1/1 -> Manual Switch2/1
  Manual Switch4/1 -> Discrete Transfer Fcn (with initial outputs)3/1, Mux3/2
  Sum/1 -> Manual Switch3/1
  Sum2/1 -> Gain/1
  Step5/1 -> Sum2/1
  Step6/1 -> Sum2/2
  setpoint velocity controller/1(V_bar_out) -> Manual Switch4/1, "Rate Limiter for fly over test "/1
  "Rate Limiter for fly over test "/1 -> Manual Switch4/2
  From File2/1 -> Manual Switch1/1
  Gain/1 -> Manual Switch3/2

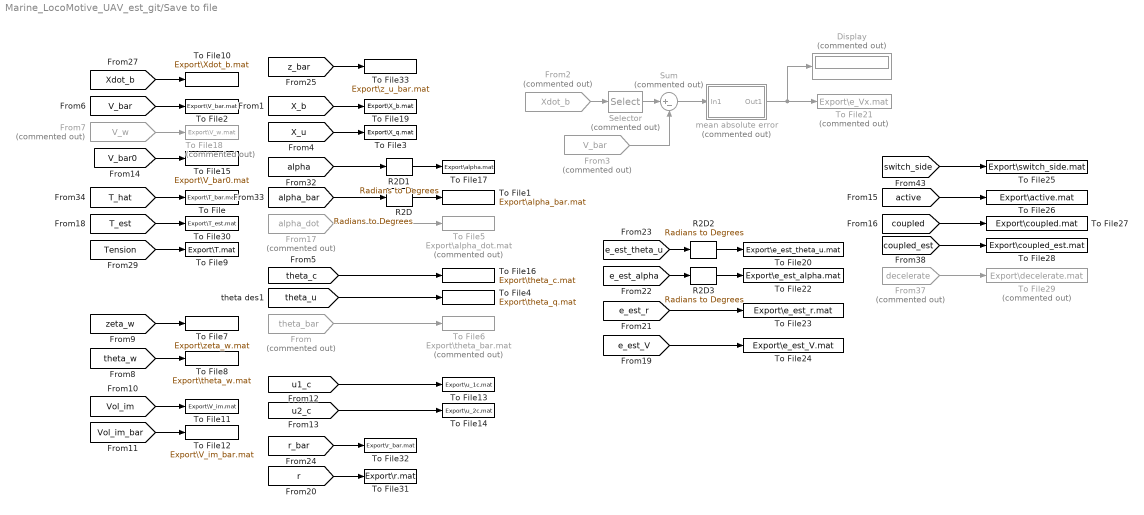
== system Marine_LocoMotive_UAV_est_git/Save to file ==
  Display : Display  Commented=on
  From : From  Commented=on  GotoTag=theta_bar  TagVisibility=global
  From17 : From  Commented=on  GotoTag=alpha_dot  TagVisibility=global
  From2 : From  Commented=on  GotoTag=Xdot_b  TagVisibility=global
  From3 : From  Commented=on  GotoTag=V_bar  TagVisibility=global
  From37 : From  Commented=on  GotoTag=decelerate  TagVisibility=global
  From7 : From  Commented=on  GotoTag=V_w  TagVisibility=global
  R2D{,1..3} (4 alike) : simulink_extras/Transformations/Radians to Degrees
  Selector : Selector  Commented=on  InputPortWidth=2  IndexOptions=Index vector (dialog)  Indices=1  OutputSizes=1
  Sum : Sum  Commented=on  Inputs=|+-
  To File : ToFile  Filename=Export\T_bar.mat  MatrixName=T_bar  SaveFormat=Timeseries  SampleTime=floor(T/4)
  To File1 : ToFile  Filename=Export\alpha_bar.mat  MatrixName=alpha_bar  SaveFormat=Timeseries  SampleTime=floor(T/4)
  To File10 : ToFile  Filename=Export\Xdot_b.mat  MatrixName=Xdot_b  SaveFormat=Timeseries  SampleTime=floor(T/4)
  To File11 : ToFile  Filename=Export\V_im.mat  MatrixName=V_im  SaveFormat=Timeseries  SampleTime=floor(T/4)
  To File12 : ToFile  Filename=Export\V_im_bar.mat  MatrixName=V_im_bar  SaveFormat=Timeseries  SampleTime=floor(T/4)
  To File13 : ToFile  Filename=Export\u_1c.mat  MatrixName=u_1c  SaveFormat=Timeseries  SampleTime=floor(T/4)
  To File14 : ToFile  Filename=Export\u_2c.mat  MatrixName=u_2c  SaveFormat=Timeseries  SampleTime=floor(T/4)
  To File15 : ToFile  Filename=Export\V_bar0.mat  MatrixName=V_bar0  SaveFormat=Timeseries  SampleTime=floor(T/4)
  To File16 : ToFile  Filename=Export\theta_c.mat  MatrixName=theta_c  SaveFormat=Timeseries  SampleTime=floor(T/4)
  To File17 : ToFile  Filename=Export\alpha.mat  MatrixName=alpha  SaveFormat=Timeseries  SampleTime=floor(T/4)
  To File18 : ToFile  Commented=on  Filename=Export\V_w.mat  MatrixName=V_w  SaveFormat=Timeseries  SampleTime=floor(T/4)
  To File19 : ToFile  Filename=Export\X_b.mat  MatrixName=X_b  SaveFormat=Timeseries  SampleTime=floor(T/4)
  To File2 : ToFile  Filename=Export\V_bar.mat  MatrixName=V_bar  SaveFormat=Timeseries  SampleTime=floor(T/4)
  To File20 : ToFile  Filename=Export\e_est_theta_u.mat  MatrixName=e_est_theta_u  SaveFormat=Timeseries  SampleTime=floor(T/4)
  To File21 : ToFile  Commented=on  Filename=Export\e_Vx.mat  MatrixName=Vx  SaveFormat=Timeseries  SampleTime=floor(T/4)
  To File22 : ToFile  Filename=Export\e_est_alpha.mat  MatrixName=e_est_alpha  SaveFormat=Timeseries  SampleTime=floor(T/4)
  To File23 : ToFile  Filename=Export\e_est_r.mat  MatrixName=e_est_r  SaveFormat=Timeseries  SampleTime=floor(T/4)
  To File24 : ToFile  Filename=Export\e_est_V.mat  MatrixName=e_est_V  SaveFormat=Timeseries  SampleTime=floor(T/4)
  To File25 : ToFile  Filename=Export\switch_side.mat  MatrixName=switch_side  SaveFormat=Timeseries  SampleTime=floor(T/4)
  To File26 : ToFile  Filename=Export\active.mat  MatrixName=active  SaveFormat=Timeseries  SampleTime=floor(T/4)
  To File27 : ToFile  Filename=Export\coupled.mat  MatrixName=coupled  SaveFormat=Timeseries  SampleTime=floor(T/4)
  To File28 : ToFile  Filename=Export\coupled_est.mat  MatrixName=coupled_est  SaveFormat=Timeseries  SampleTime=floor(T/4)
  To File29 : ToFile  Commented=on  Filename=Export\decelerate.mat  MatrixName=decelerate  SaveFormat=Timeseries  SampleTime=floor(T/4)
  To File3 : ToFile  Filename=Export\X_q.mat  MatrixName=X_q  SaveFormat=Timeseries  SampleTime=floor(T/4)
  To File30 : ToFile  Filename=Export\T_est.mat  MatrixName=T_est  SaveFormat=Timeseries  SampleTime=floor(T/4)
  To File31 : ToFile  Filename=Export\r.mat  MatrixName=r  SaveFormat=Timeseries  SampleTime=floor(T/4)
  To File32 : ToFile  Filename=Export\r_bar.mat  MatrixName=r_bar  SaveFormat=Timeseries  SampleTime=floor(T/4)
  To File33 : ToFile  Filename=Export\z_u_bar.mat  MatrixName=z_u_bar  SaveFormat=Timeseries  SampleTime=floor(T/4)
  To File4 : ToFile  Filename=Export\theta_q.mat  MatrixName=theta_q  SaveFormat=Timeseries  SampleTime=floor(T/4)
  To File5 : ToFile  Commented=on  Filename=Export\alpha_dot.mat  MatrixName=alpha_dot  SaveFormat=Timeseries  SampleTime=floor(T/4)
  To File6 : ToFile  Commented=on  Filename=Export\theta_bar.mat  MatrixName=theta_bar  SaveFormat=Timeseries  SampleTime=floor(T/4)
  To File7 : ToFile  Filename=Export\zeta_w.mat  MatrixName=zeta_w  SaveFormat=Timeseries  SampleTime=floor(T/4)
  To File8 : ToFile  Filename=Export\theta_w.mat  MatrixName=theta_w  SaveFormat=Timeseries  SampleTime=floor(T/4)
  To File9 : ToFile  Filename=Export\T.mat  MatrixName=T  SaveFormat=Timeseries  SampleTime=floor(T/4)
  mean absolute error : Subsystem  Commented=on
  wires:
  R2D/1 -> To File1/1
  [X_u] -> To File3/1
  [alpha_bar] -> R2D/1
  [V_bar] -> To File2/1
  [theta_c] -> To File16/1
  [alpha] -> R2D1/1
  R2D1/1 -> To File17/1
  From7/1 -> To File18/1
  [X_b] -> To File19/1
  Sum/1 -> mean absolute error/1(In1)
  mean absolute error/1(Out1) -> Display/1, To File21/1
  [T_hat] -> To File/1
  [theta_u] -> To File4/1
  From17/1 -> To File5/1
  From/1 -> To File6/1
  [zeta_w] -> To File7/1
  [theta_w] -> To File8/1
  [Tension] -> To File9/1
  [Xdot_b] -> To File10/1
  From2/1 -> Selector/1
  From3/1 -> Sum/2
  Selector/1 -> Sum/1
  [Vol_im] -> To File11/1
  [Vol_im_bar] -> To File12/1
  [u1_c] -> To File13/1
  [u2_c] -> To File14/1
  [V_bar0] -> To File15/1
  [e_est_theta_u] -> R2D2/1
  R2D2/1 -> To File20/1
  [e_est_alpha] -> R2D3/1
  R2D3/1 -> To File22/1
  [e_est_r] -> To File23/1
  [e_est_V] -> To File24/1
  [switch_side] -> To File25/1
  [active] -> To File26/1
  [coupled] -> To File27/1
  [coupled_est] -> To File28/1
  From37/1 -> To File29/1
  [T_est] -> To File30/1
  [r] -> To File31/1
  [r_bar] -> To File32/1
  [z_bar] -> To File33/1

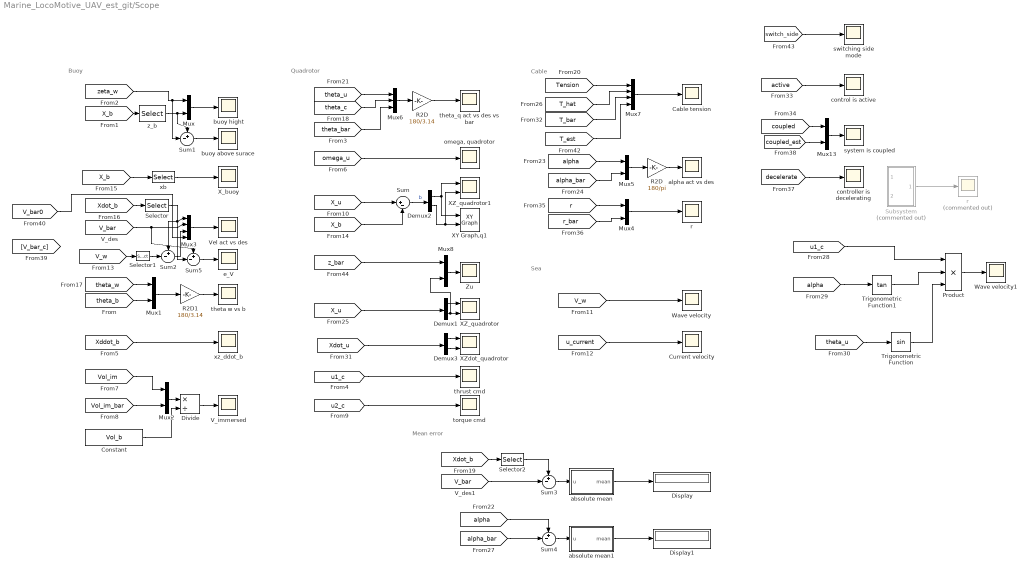
== system Marine_LocoMotive_UAV_est_git/Scope ==
  note: Mean error
  note: Sea
  note: Cable
  note: Quadrotor
  note: Buoy
  " r" : Scope
  Cable tension : Scope
  Constant : Constant  Value=Vol_b
  Current velocity : Scope
  Demux1 : Demux  Outputs=2
  Demux2 : Demux  Outputs=2
  Demux3 : Demux  Outputs=2
  Display : Display
  Display1 : Display
  Divide : Product  Inputs=*/
  Mux{,1..2,4..5,8,13} (7 alike) : Mux  Inputs=2
  Mux3 : Mux
  Mux6 : Mux  Inputs=3
  Mux7 : Mux
  Product : Product  Inputs=3
  R2D : Gain  Gain=180/3.14
  "R2D " : Gain  Gain=180/pi
  R2D1 : Gain  Gain=180/3.14
  Selector : Selector  InputPortWidth=2  IndexOptions=Index vector (dialog)  Indices=1  OutputSizes=1
  Selector1 : Selector  InputPortWidth=2  IndexOptions=Index vector (dialog)  Indices=1  OutputSizes=1
  Selector2 : Selector  InputPortWidth=2  IndexOptions=Index vector (dialog)  Indices=1  OutputSizes=1
  Subsystem : Subsystem  Commented=on
  Sum : Sum  Inputs=|+-
  Sum{1..5} (5 alike) : Sum  Inputs=+-|
  Trigonometric Function : Trigonometry
  Trigonometric Function1 : Trigonometry  Operator=tan
  V_immersed : Scope
  Vel act vs des : Scope
  Wave velocity : Scope
  Wave velocity1 : Scope
  XY Graph,q1 : simulink/Sinks/XY Graph  xmin=-17  xmax=17  ymin=0  ymax=17  st=1/10
  XZ_quadrotor : Scope  NumInputPorts=2
  XZ_quadrotor1 : Scope  NumInputPorts=2
  XZdot_quadrotor : Scope  NumInputPorts=2
  X_buoy : Scope
  Zu : Scope
  absolute mean : Subsystem
  absolute mean1 : Subsystem
  "alpha act vs des " : Scope
  buoy above surace : Scope
  buoy hight : Scope
  control is active : Scope
  controller is decelerating : Scope
  e_V : Scope
  "omega, quadrotor" : Scope
  r : Scope  Commented=on
  switching side mode : Scope
  system is coupled : Scope
  theta w vs b : Scope
  theta_q act vs des vs bar : Scope
  thrust cmd : Scope
  torque cmd : Scope
  xb : Selector  InputPortWidth=2  IndexOptions=Index vector (dialog)  Indices=1  OutputSizes=1
  xz_ddot_b : Scope
  z_b : Selector  InputPortWidth=2  IndexOptions=Index vector (dialog)  Indices=2  OutputSizes=1
  wires:
  Mux/1 -> buoy hight/1
  z_b/1 -> Sum1/1, Mux/2
  [zeta_w] -> Sum1/2, Mux/1
  [omega_u] -> "omega, quadrotor"/1
  [X_b] -> Sum/2
  Sum/1 -> Demux2/1  "b"
  [X_b] -> z_b/1
  Sum1/1 -> buoy above surace/1
  Mux1/1 -> R2D1/1
  Mux6/1 -> R2D/1
  Mux7/1 -> Cable tension/1
  Demux2/2 -> XZ_quadrotor1/2, XY Graph,q1/2
  Demux2/1 -> XZ_quadrotor1/1, XY Graph,q1/1
  [V_bar] -> Sum5/1, Mux3/2
  [Xdot_b] -> Selector/1
  [theta_c] -> Mux6/2
  [theta_u] -> Mux6/1
  Mux3/1 -> Vel act vs des/1
  [alpha] -> Mux5/1
  [alpha_bar] -> Mux5/2
  Mux5/1 -> "R2D "/1
  [X_u] -> Sum/1
  [X_u] -> Demux1/1
  Selector/1 -> Sum5/2, Sum2/1, Mux3/1
  "R2D "/1 -> "alpha act vs des "/1
  [Tension] -> Mux7/1
  [T_hat] -> Mux7/2
  [theta_b] -> Mux1/2
  [theta_w] -> Mux1/1
  Subsystem/1(Out1) -> r/1
  [theta_bar] -> Mux6/3
  R2D/1 -> theta_q act vs des vs bar/1
  [X_b] -> xb/1
  xb/1 -> X_buoy/1
  [Xddot_b] -> xz_ddot_b/1
  [Vol_im] -> Mux2/1
  [Vol_im_bar] -> Mux2/2
  Divide/1 -> V_immersed/1
  R2D1/1 -> theta w vs b/1
  Mux2/1 -> Divide/1
  Constant/1 -> Divide/2
  [u1_c] -> thrust cmd/1
  [u2_c] -> torque cmd/1
  [V_w] -> Wave velocity/1
  [u_current] -> Current velocity/1
  Demux1/2 -> Mux8/2, XZ_quadrotor/2
  Demux1/1 -> XZ_quadrotor/1
  [V_w] -> Selector1/1
  Sum2/1 -> Mux3/3
  Selector1/1 -> Sum2/2
  [Xdot_b] -> Selector2/1
  [V_bar] -> Sum3/2
  Selector2/1 -> Sum3/1
  Sum3/1 -> absolute mean/1(u)
  absolute mean/1(mean) -> Display/1
  [alpha] -> Sum4/1
  [alpha_bar] -> Sum4/2
  Sum4/1 -> absolute mean1/1(u)
  absolute mean1/1(mean) -> Display1/1
  [alpha] -> Trigonometric Function1/1
  [theta_u] -> Trigonometric Function/1
  [u1_c] -> Product/1
  Trigonometric Function1/1 -> Product/2
  Trigonometric Function/1 -> Product/3
  Product/1 -> Wave velocity1/1
  [T_bar] -> Mux7/3
  Demux3/2 -> XZdot_quadrotor/2
  [Xdot_u] -> Demux3/1
  Demux3/1 -> XZdot_quadrotor/1
  [active] -> control is active/1
  [coupled] -> Mux13/1
  [r] -> Mux4/1
  Mux4/1 -> " r"/1
  [r_bar] -> Mux4/2
  [decelerate] -> controller is decelerating/1
  [coupled_est] -> Mux13/2
  Mux13/1 -> system is coupled/1
  Sum5/1 -> e_V/1
  [z_bar] -> Mux8/1
  Mux8/1 -> Zu/1
  [T_est] -> Mux7/4
  [switch_side] -> switching side mode/1
  [V_bar0] -> Mux3/4

== system Marine_LocoMotive_UAV_est_git/Sea2 ==
  note: Water elevation at buoy location (x_b)
  note: Total Current (without stocks drift)
  note: Water elevation at buoy location (x_b)
  X_b : Inport
  time : Inport  Port=2
  " current" : Scope
  Add : Sum  Inputs=2
  Constant1 : Constant  Value=H
  Constant2 : Constant  Value=H
  Gain1 : Gain  Gain=k_w
  Gain2 : Gain  Gain=k_w2
  Math Function1 : Math  SaturateOnIntegerOverflow=on
  Math Function2 : Math  SaturateOnIntegerOverflow=on
  Mean water level : Bias  Bias=H
  Product{1..4} (4 alike) : Product
  Single Wave : Subsystem  mask(Wave Model){A=A_w, omega=omega_w, k=k_w, epsilon=epsilon_w, w_dir=w_dir}
      mask prompts: A "Wave amplitude, A (m):"; omega "Circular frequency (rad):"; k "wave number, k:"; epsilon "Random phase angle (rad):"; w_dir "Wave direction:"
      mask help: Wave Model for a single wave in 2D.
      mask Display:
      | port_label('input',1,'t (s)','texmode','on');
      | port_label('input',2,'x(t) (m)','texmode','on');
      | 
      | port_label('output',1,'\zeta (x,t)','texmode','on');
      | port_label('output',2,'\theta_{w} (x,t)','texmode','on');
      | port_label('output',3,'u(z_0,x,t) (m/s)','texmode','on');
      | port_label('output',4,'w(z_0,x,t) (m/s)','texmode','on');
  Single Wave1 : Subsystem  mask(Wave Model){A=A_w2, omega=omega_w2, k=k_w2, epsilon=epsilon_w2, w_dir=w_dir2}
      mask prompts: A "Wave amplitude, A (m):"; omega "Circular frequency (rad):"; k "wave number, k:"; epsilon "Random phase angle (rad):"; w_dir "Wave direction:"
      mask help: Wave Model for a single wave in 2D.
      mask Display:
      | port_label('input',1,'t (s)','texmode','on');
      | port_label('input',2,'x(t) (m)','texmode','on');
      | 
      | port_label('output',1,'\zeta (x,t)','texmode','on');
      | port_label('output',2,'\theta_{w} (x,t)','texmode','on');
      | port_label('output',3,'u(z_0,x,t) (m/s)','texmode','on');
      | port_label('output',4,'w(z_0,x,t) (m/s)','texmode','on');
  Sum1 : Sum  Inputs=|++
  Sum{2,4..5,7..8} (5 alike) : Sum  Inputs=++|
  Sum3 : Sum  Inputs=|+-
  Sum6 : Sum  Inputs=|+-
  Theta_water surface (two waves) : Subsystem
  Trigonometric Function1 : Trigonometry  Operator=atan
  Vector Concatenate : Concatenate
  Vector Concatenate1 : Concatenate
  Vector Concatenate2 : Concatenate
  stocks drift1 : Constant  Value=u_s
  stocks drift2 : Constant  Value=u_s2
  tidal current : Constant  Value=u_t
  u : Scope
  u2 : Scope
  w : Scope
  w1 : Scope
  w2 : Scope
  wind generated current : Constant  Value=u_w
  x_b : Selector  InputPortWidth=2  IndexOptions=Index vector (dialog)  Indices=1  OutputSizes=1
  z_b : Selector  InputPortWidth=2  IndexOptions=Index vector (dialog)  Indices=2  OutputSizes=1
  z_b1 : Selector  InputPortWidth=2  IndexOptions=Index vector (dialog)  Indices=2  OutputSizes=1
  zeta(x,t) : Outport
  v_xz(x,t) : Outport  Port=2
  theta_w : Outport  Port=3
  u_cur : Outport  Port=4
  wires:
  z_b/1 -> Sum3/1
  tidal current/1 -> Add/1
  wind generated current/1 -> Add/2
  Sum1/1 -> u/1, Vector Concatenate/1
  Add/1 -> u_cur/1, " current"/1, Sum1/2  "Ut.x"
  Vector Concatenate/1 -> Sum8/2
  Constant1/1 -> Sum3/2
  Single Wave/2(theta_w(x,t)) -> Sum5/2
  time/1 -> Single Wave1/1(time), Single Wave/1(time)
  x_b/1 -> Single Wave1/2(x(t)), Single Wave/2(x(t))
  Sum3/1 -> Gain1/1
  stocks drift1/1 -> Sum4/1  "u_bar (transport velocity)"
  Math Function1/1 -> Product1/2, Product3/2  "decay"
  Sum4/1 -> Sum1/1
  Product1/1 -> Sum4/2  "u(x,t)"
  Gain1/1 -> Math Function1/1
  Single Wave/1(zeta(x,t)) -> Sum2/2
  Product3/1 -> w/1, Vector Concatenate/2
  Mean water level/1 -> zeta(x,t)/1
  Single Wave/3(u(z0,x,t)) -> Product1/1
  Single Wave/4(w(z0,x,t)) -> Theta_water surface (two waves)/1(w1), Product3/1
  Trigonometric Function1/1 -> Vector Concatenate1/1, theta_w/1
  Vector Concatenate1/1 -> u2/1
  Theta_water surface (two waves)/1(Out1) -> Trigonometric Function1/1
  Single Wave1/1(zeta(x,t)) -> Sum2/1
  Single Wave1/2(theta_w(x,t)) -> Sum5/1
  Sum5/1 -> Vector Concatenate1/2
  Sum2/1 -> Mean water level/1
  Sum6/1 -> Gain2/1
  z_b1/1 -> Sum6/1
  X_b/1 -> z_b1/1, x_b/1, z_b/1
  Gain2/1 -> Math Function2/1
  Constant2/1 -> Sum6/2
  Single Wave1/4(w(z0,x,t)) -> Product4/1, Theta_water surface (two waves)/2(w2)
  Single Wave1/3(u(z0,x,t)) -> Product2/1
  Product4/1 -> w2/1, Vector Concatenate2/2
  Product2/1 -> Sum7/2  "u(x,t)"
  Math Function2/1 -> Product4/2, Product2/2  "decay"
  stocks drift2/1 -> Sum7/1
  Sum7/1 -> Vector Concatenate2/1
  Vector Concatenate2/1 -> Sum8/1
  Sum8/1 -> w1/1, v_xz(x,t)/1
